simulink model "exampleIPCore"  (R2024a)
settings: Solver=FixedStepDiscrete  StartTime=0.0  StopTime=10.0  RelTol=1e-3
settings Model: DataTypeOverride=Off  Creator=cotti  LastModifiedBy=cotti
settings OptimizationCC: BlockReduction=off  ConditionallyExecuteInputs=off  DefaultParameterBehavior=Inlined  InheritOutputTypeSmallerThanSingle=on
settings DebuggingCC: AlgebraicLoopMsg=error  SingleTaskRateTransMsg=error  UnconnectedInputMsg=warning  UnconnectedOutputMsg=warning  UnconnectedLineMsg=warning
settings HardwareCC: ProdBitPerPointer=32  ProdBitPerSizeT=32  ProdBitPerPtrDiffT=32  ProdLargestAtomicFloat=None  ProdIntDivRoundTo=Undefined  ProdEndianess=Unspecified  ProdWordSize=32  ProdHWDeviceType=ASIC/FPGA->ASIC/FPGA  TargetBitPerLong=64  TargetBitPerPointer=64  TargetBitPerSizeT=64  TargetBitPerPtrDiffT=64  TargetLongLongMode=on  TargetIntDivRoundTo=Zero  TargetEndianess=LittleEndian  TargetWordSize=64  TargetHWDeviceType=Custom Processor->MATLAB Host Computer  ProdEqTarget=off

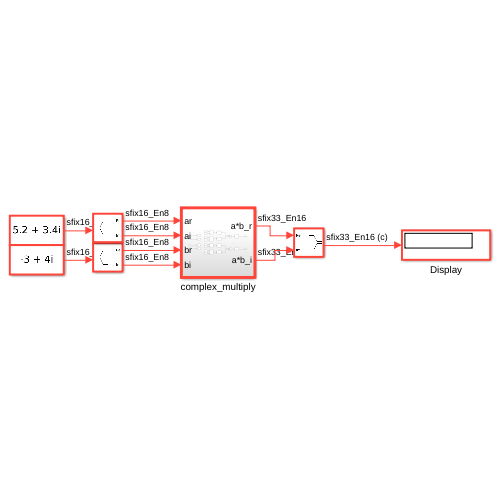
[thumbnail: Simulink's stored preview of the top-level diagram]
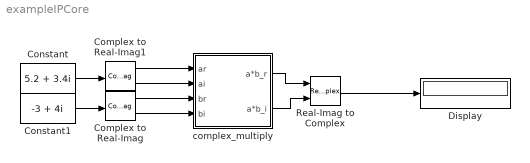
== system exampleIPCore ==
  Complex to Real-Imag : ComplexToRealImag
  Complex to Real-Imag1 : ComplexToRealImag
  Constant : Constant  Value=5.2 + 3.4i  OutDataTypeStr=fixdt(1,16,8)  SampleTime=-1
  Constant1 : Constant  Value=-3 + 4i  OutDataTypeStr=fixdt(1,16,8)  SampleTime=-1
  Display : Display
  Real-Imag to Complex : RealImagToComplex
  complex_multiply : Subsystem  TreatAsAtomicUnit=on
  wires:
  Constant1/1 -> Complex to Real-Imag/1
  Constant/1 -> Complex to Real-Imag1/1
  Complex to Real-Imag1/1 -> complex_multiply/1(ar)
  Complex to Real-Imag1/2 -> complex_multiply/2(ai)
  Complex to Real-Imag/1 -> complex_multiply/3(br)
  Complex to Real-Imag/2 -> complex_multiply/4(bi)
  complex_multiply/1(a*b_r) -> Real-Imag to Complex/1
  complex_multiply/2(a*b_i) -> Real-Imag to Complex/2
  Real-Imag to Complex/1 -> Display/1

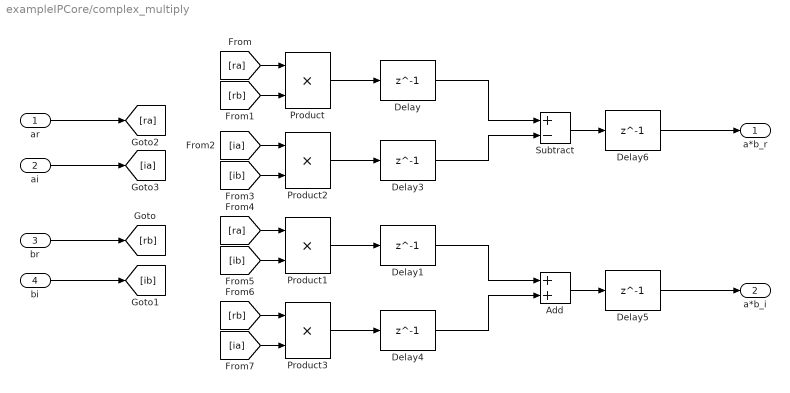
== system exampleIPCore/complex_multiply ==
  ar : Inport
  ai : Inport  Port=2
  br : Inport  Port=3
  bi : Inport  Port=4
  Add : Sum
  Delay{,1,3..6} (6 alike) : Delay  DelayLength=1  InitialCondition=0  UseCircularBuffer=on
  Product{,1..3} (4 alike) : Product
  Subtract : Sum  Inputs=+-
  a*b_r : Outport
  a*b_i : Outport  Port=2
  wires:
  Product/1 -> Delay/1
  br/1 -> [rb]
  bi/1 -> [ib]
  ar/1 -> [ra]
  ai/1 -> [ia]
  [ra] -> Product/1
  [rb] -> Product/2
  [ib] -> Product2/2
  Product2/1 -> Delay3/1
  [ia] -> Product2/1
  Product1/1 -> Delay1/1
  [ib] -> Product1/2
  [ra] -> Product1/1
  Product3/1 -> Delay4/1
  [ia] -> Product3/2
  [rb] -> Product3/1
  Delay1/1 -> Add/1
  Delay4/1 -> Add/2
  Add/1 -> Delay5/1
  Subtract/1 -> Delay6/1
  Delay/1 -> Subtract/1
  Delay3/1 -> Subtract/2
  Delay6/1 -> a*b_r/1
  Delay5/1 -> a*b_i/1
